simulink model "sampleModel299"  (R2021b)
settings: Solver=VariableStepAuto  StartTime=0.0  StopTime=10.0  RelTol=1e-3
libraries: simulink x4
settings Model: Creator=user  LastModifiedBy=user

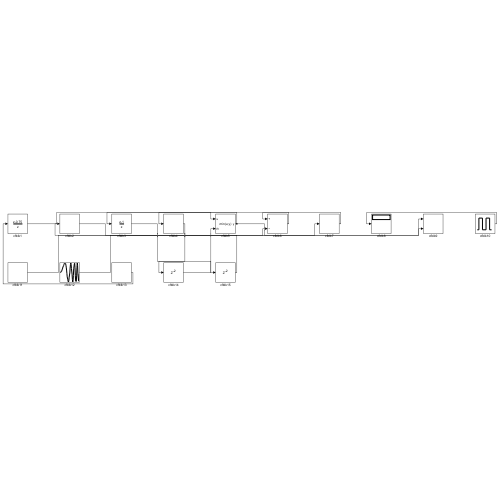
[thumbnail: Simulink's stored preview of the top-level diagram]
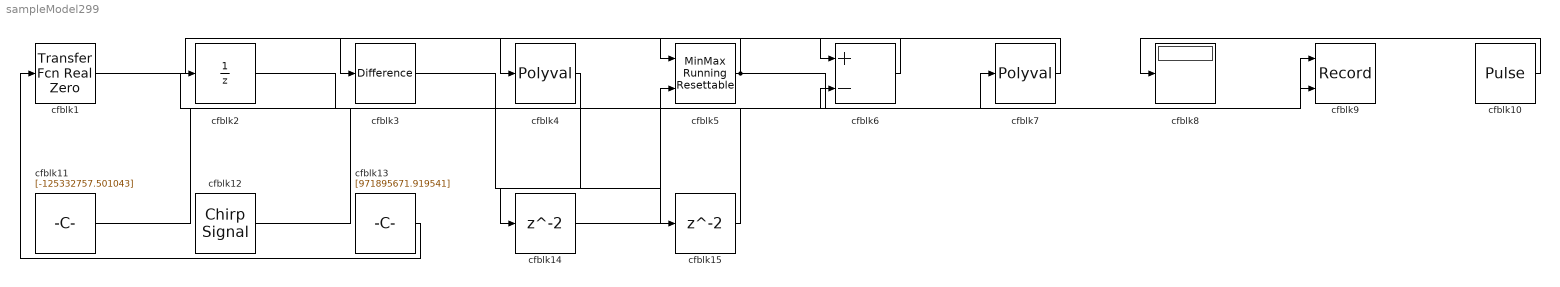
== system sampleModel299 ==
  cfblk1 : simulink/Discrete/Transfer Fcn Real Zero  ZeroZ=0.75  ICPrevInput=0.0  DoSatur=off
      settings: SourceProductBaseCode=SL
  cfblk10 : DiscretePulseGenerator  PulseType=Time based  Amplitude=[684580611.940352]  Period=[90863037.478560]  PulseWidth=5  PhaseDelay=[5.000000]
  cfblk11 : Constant  Value=[-125332757.501043]  SampleTime=1
  cfblk12 : simulink/Sources/Chirp Signal  f1=[439640241.666335]  T=[-443937567.420057]  f2=[-682344816.743202]
  cfblk13 : Constant  Value=[971895671.919541]  SampleTime=1
  cfblk14 : Delay  SampleTime=1
  cfblk15 : Delay  SampleTime=1
  cfblk2 : UnitDelay  HasFrameUpgradeWarning=on
  cfblk3 : simulink/Discrete/Difference  ICPrevInput=0.0  OutMin=[]  OutMax=[]  OutDataTypeStr=Inherit: Inherit via back propagation  OutDataType=fixdt(1, 16)  OutScaling=2^-10  DoSatur=off
  cfblk4 : Polyval  Coefs=[ +2.081618890e-019, -1.441693666e-014, +4.719686976e-010, -8.536869453e-006, +1.621573104e-001, -8.087801117e+001 ]
  cfblk5 : simulink/Math Operations/MinMax Running Resettable  Function=min  vinit=0.0
  cfblk6 : Sum  Inputs=+-
  cfblk7 : Polyval  Coefs=[ +2.081618890e-019, -1.441693666e-014, +4.719686976e-010, -8.536869453e-006, +1.621573104e-001, -8.087801117e+001 ]
  cfblk8 : Display
  cfblk9 : Record  FileSettingsInternal="{\"entries\":[{\"content\":{\"excelSettings\":{\"content\":{},\"type\":\"Streamout.ExcelSettings\"}},\"type\":\"Streamout.FileSettingStorage\",\"uuid\":\"9b7841ad-6a22-4a8e-a1cf-05eca4c7cefb\"}],\"packageUris\":[\"http://schema.mathworks.com/mf0/streamout_blocks/R2020a\"],\"version\":\"1.0\"}"  Layout=[1 1]  SignalsInternal="{\"entries\":[{\"content\":{\"signals\":[{\"content\":{\"blockPath\":[\"sampleModel299/cfblk9\"],\"channel\":[],\"dimensions\":[1],\"domain\":\"sampleModel299/cfblk9\",\"lineColor\":\"#a2142f\",\"plots\":[1],\"port\":1,\"sid\":[\"\"],\"signalID\":12898,\"signalName\":\"cfblk11\"},\"type\":\"RecordBlkView.Signal\",\"uuid\":\"0ef4b418-99a9-4e30-9209-0d92b90a0cbb\"},{\"content\":{\"blockPath\":[\"sampleModel299/cfblk9\"],\"channel\":[],\"dimensions\":[1],\"domain\":\"sampleModel299/cfblk9\",\"lineColor\":\"#139fff\",\"plots\":[1],\"port\":2,\"sid\":[\"\"],\"signalID\":12902,\"signalName\":\"cfblk5\"},\"type\":\"RecordBlkView.Signal\",\"uuid\":\"0a2f009f-081b-4d03-aa2c-4dd6f11cf530\"}]},\"type\":\"RecordBlkView.InputSignals\",\"uuid\":\"d84d1abe-e92a-4215-93ad-a0061b9bedec\"}],\"packageUris\":[\"http://schema.mathworks.com/mf0/streamout_blocks/R2020a\"],\"version\":\"1.0\"}"  VisualizationBindings="{\"xyplotplugin\":{\"info\":[{\"series\":[{\"bindingParametersList\":[{\"parameter\":\"X-Axis\",\"signalID\":12898,\"signalName\":\"cfblk11\"},{\"parameter\":\"Y-Axis\",\"signalID\":12902,\"signalName\":\"cfblk5\"}],\"seriesID\":53874}],\"subplotID\":1}]}}"  CompatibilityTag=XY
  wires:
  cfblk11/1 -> cfblk9/1
  cfblk5/1 -> cfblk9/2, cfblk4/1
  cfblk1/1 -> cfblk5/1
  cfblk13/1 -> cfblk1/1
  cfblk6/1 -> cfblk3/1
  cfblk7/1 -> cfblk6/1
  cfblk12/1 -> cfblk7/1
  cfblk2/1 -> cfblk6/2
  cfblk10/1 -> cfblk8/1
  cfblk4/1 -> cfblk14/1
  cfblk14/1 -> cfblk5/2
  cfblk3/1 -> cfblk15/1
  cfblk15/1 -> cfblk2/1
